simulink model "case_5_cut_in25a"  (R2025a)
settings: Solver=VariableStepAuto  StartTime=0.0  StopTime=10.0  RelTol=1e-3
settings Model: Creator=jdcjd  LastModifiedBy=jdcjd

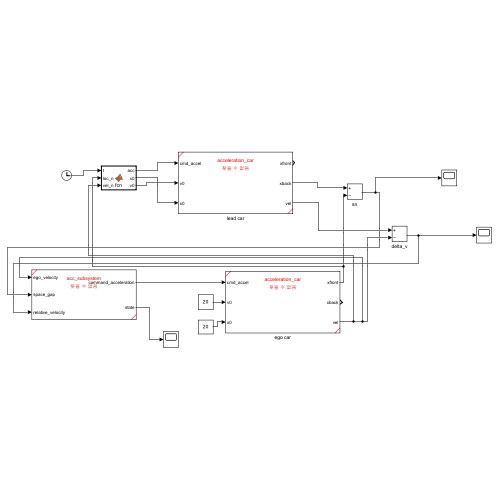
[thumbnail: Simulink's stored preview of the top-level diagram]
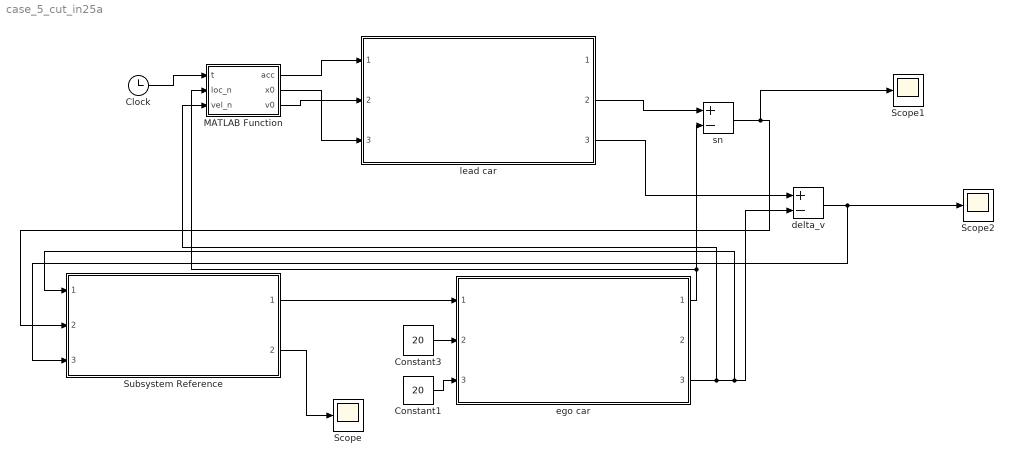
== system case_5_cut_in25a ==
  Clock : Clock
  Constant1 : Constant  Value=20
  Constant3 : Constant  Value=20
  MATLAB Function : MATLAB Function  TreatAsAtomicUnit=on
  Scope : Scope
  Scope1 : Scope
  Scope2 : Scope
      settings: DataLoggingVariableName=ScopeData2
  Subsystem Reference : Subsystem  ReferencedSubsystem=acc_subsystem
  delta_v : Sum  Inputs=+-
  ego car : Subsystem  ReferencedSubsystem=acceleration_car
  lead car : Subsystem  ReferencedSubsystem=acceleration_car
  sn : Sum  Inputs=+-
  wires:
  lead car/2 -> sn/1
  ego car/1 -> MATLAB Function/2(loc_n), sn/2
  lead car/3 -> delta_v/1
  ego car/3 -> MATLAB Function/3(vel_n), Subsystem Reference/1, delta_v/2
  Subsystem Reference/1 -> ego car/1
  sn/1 -> Scope1/1, Subsystem Reference/2
  delta_v/1 -> Scope2/1, Subsystem Reference/3
  Subsystem Reference/2 -> Scope/1
  Constant3/1 -> ego car/2
  Constant1/1 -> ego car/3
  Clock/1 -> MATLAB Function/1(t)
  MATLAB Function/1(acc) -> lead car/1
  MATLAB Function/2(x0) -> lead car/3
  MATLAB Function/3(v0) -> lead car/2

== matlab function case_5_cut_in25a/MATLAB Function ==
  data: t input; acc output; loc_n input; vel_n input; x0 output; v0 output
function [acc, x0, v0] = fcn(t, loc_n, vel_n)

if t < 5
    acc = 0;
    x0 = 0;
    v0 = 0;
else 
    acc = 1;
    x0 = loc_n + 5;
    v0 = vel_n;

end
end
